simulink model "tank_thermal_sensor_comparison"  (R2025b)
settings: Solver=ode45  StartTime=0.0  StopTime=3600  RelTol=1e-3
libraries: slpidlib x1
settings Model: Creator=maild  LastModifiedBy=maild

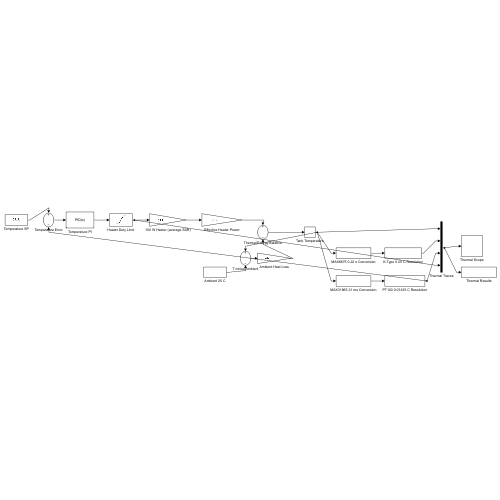
[thumbnail: Simulink's stored preview of the top-level diagram]
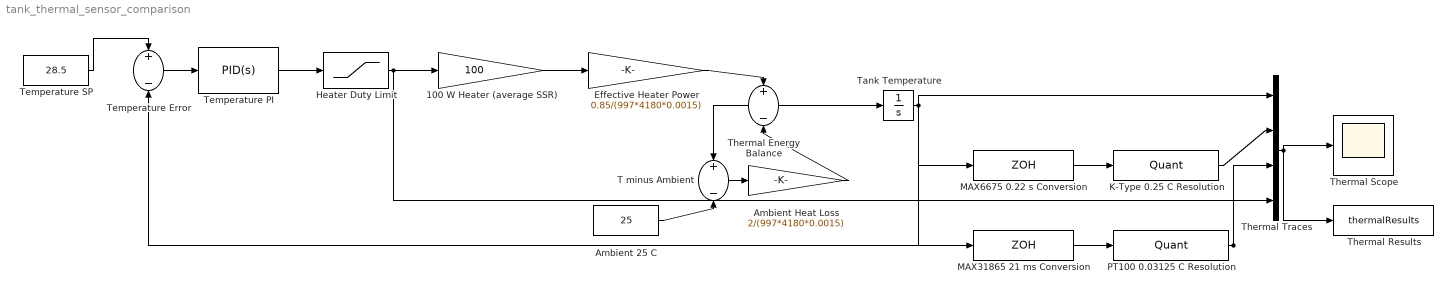
== system tank_thermal_sensor_comparison ==
  100 W Heater (average SSR) : Gain  Gain=100
  Ambient 25 C : Constant  Value=25
  Ambient Heat Loss : Gain  Gain=2/(997*4180*0.0015)
  Effective Heater Power : Gain  Gain=0.85/(997*4180*0.0015)
  Heater Duty Limit : Saturate  UpperLimit=0.10  LowerLimit=0
  K-Type 0.25 C Resolution : Quantizer  QuantizationInterval=0.25
  MAX31865 21 ms Conversion : ZeroOrderHold  SampleTime=0.021
  MAX6675 0.22 s Conversion : ZeroOrderHold  SampleTime=0.22
  PT100 0.03125 C Resolution : Quantizer  QuantizationInterval=0.03125
  T minus Ambient : Sum  Inputs=+-
  Tank Temperature : Integrator  InitialCondition=25
  Temperature Error : Sum  Inputs=+-
  Temperature PI : slpidlib/PID Controller  Controller=PID  Form=Parallel  TimeDomain=Continuous-time  UseExternalTs=off  SampleTime=-1  IntegratorMethod=Forward Euler  FilterMethod=Forward Euler  ControllerParametersSource=internal  P=0.04  I=0.0008  UseKiTs=off  D=0  UseExternalDerivativeSource=off  N=100  UseFilter=on  TunerSelectOption=Transfer Function Based (PID Tuner App)  InitialConditionSource=internal  InitialConditionForIntegrator=0  InitialConditionForFilter=0  DifferentiatorICPrevScaledInput=0  ExternalReset=none  TrackingMode=off  Kt=1  LimitOutput=off  SatLimitsSource=internal  UpperSaturationLimit=inf  LowerSaturationLimit=-inf  LinearizeAsGain=on  AntiWindupMode=none  Kb=1  LimitIntegrator=off  UpperIntegratorSaturationLimit=inf  LowerIntegratorSaturationLimit=-inf  POutMin=[]  POutMax=[]  IOutMin=[]  IOutMax=[]  DOutMin=[]  DOutMax=[]  NOutMin=[]  NOutMax=[]  SumOutMin=[]  SumOutMax=[]  SaturationOutMin=[]  SaturationOutMax=[]  PParamMin=[]  PParamMax=[]  IParamMin=[]  IParamMax=[]  DParamMin=[]  DParamMax=[]  NParamMin=[]  NParamMax=[]  KbParamMin=[]  KbParamMax=[]  KtParamMin=[]  KtParamMax=[]  KbOutMin=[]  KbOutMax=[]  KtOutMin=[]  KtOutMax=[]  IntegratorOutMin=[]  IntegratorOutMax=[]  FilterOutMin=[]  FilterOutMax=[]  SumI1OutMin=[]  SumI1OutMax=[]  SumI2OutMin=[]  SumI2OutMax=[]  SumI3OutMin=[]  SumI3OutMax=[]  SumI4OutMin=[]  SumI4OutMax=[]  SumDOutMin=[]  SumDOutMax=[]  DifferentiatorOutMin=[]  DifferentiatorOutMax=[]  FilterDiffOutCoefMin=[]  FilterDiffOutCoefMax=[]  ReciprocalOutMin=[]  ReciprocalOutMax=[]  SumDenOutMin=[]  SumDenOutMax=[]  SumNumOutMin=[]  SumNumOutMax=[]  DivideOutMin=[]  DivideOutMax=[]  UdiffTsProdOutMin=[]  UdiffTsProdOutMax=[]  NTsProdOutMin=[]  NTsProdOutMax=[]  UintegralTsProdOutMin=[]  UintegralTsProdOutMax=[]  UngainTsProdOutMin=[]  UngainTsProdOutMax=[]  ClampingZeroOutDataTypeStr=Inherit: Inherit via back propagation  ClampingZeroOutMin=[]  ClampingZeroOutMax=[]  FilterDenConstantOutDataTypeStr=Inherit: Inherit via back propagation  FilterDenConstantOutMin=[]  FilterDenConstantOutMax=[]  PCopyOutDataTypeStr=Inherit: Inherit via back propagation  PCopyOutMin=[]  PCopyOutMax=[]  NCopyOutDataTypeStr=Inherit: Inherit via back propagation  NCopyOutMin=[]  NCopyOutMax=[]  IntegratorContinuousStateAttributes=''  IntegratorStateMustResolveToSignalObject=off  IntegratorRTWStateStorageClass=Auto  FilterContinuousStateAttributes=''  FilterStateMustResolveToSignalObject=off  FilterRTWStateStorageClass=Auto  ParallelPVariant=InternalParameters  IdealPVariant=Disabled  IVariant=InternalParameters  DVariant=InternalParameters  IntegratorVariant=Continuous  SatVariant=Disabled  AWVariant=Passthrough  PCopyVariant=Disabled  TRVariant=Disabled  FdbkBlocksVariant=Forward  IdealPFdbkVariant=Disabled  SatFdbkVariant=Disabled  DerivativeFilterVariant=ContFilter  NVariant=InternalParameters  NCopyVariant=Disabled  FilterICVariant=InternalICsFilter  IntegratorICVariant=InternalICs  ExternalResetVariant=Disabled  TRSumVariant=Passthrough  SumFdbkVariant=Disabled  SumVariant=Sum_PID  TsampFilterVariant=InternalTs  TsampNgainVariant=Passthrough  TsampIntegralVariant=Disabled_SignalSpec  ExternalSaturationOutDataTypeStr=Inherit: Same as second input  DerivativeSourceVariant=ErrorSignal  PreIntVariant=InternalPreInt
  Temperature SP : Constant  Value=28.5
  Thermal Energy Balance : Sum  Inputs=+-
  Thermal Results : ToWorkspace  VariableName=thermalResults  SaveFormat=Structure With Time  SampleTime=-1
  Thermal Scope : Scope
  Thermal Traces : Mux
  wires:
  Temperature SP/1 -> Temperature Error/1
  Temperature Error/1 -> Temperature PI/1
  Temperature PI/1 -> Heater Duty Limit/1
  Heater Duty Limit/1 -> 100 W Heater (average SSR)/1, Thermal Traces/4
  100 W Heater (average SSR)/1 -> Effective Heater Power/1
  Effective Heater Power/1 -> Thermal Energy Balance/1
  Tank Temperature/1 -> T minus Ambient/1, MAX6675 0.22 s Conversion/1, MAX31865 21 ms Conversion/1, Thermal Traces/1
  Ambient 25 C/1 -> T minus Ambient/2
  T minus Ambient/1 -> Ambient Heat Loss/1
  Ambient Heat Loss/1 -> Thermal Energy Balance/2
  Thermal Energy Balance/1 -> Tank Temperature/1
  MAX6675 0.22 s Conversion/1 -> K-Type 0.25 C Resolution/1
  MAX31865 21 ms Conversion/1 -> PT100 0.03125 C Resolution/1
  PT100 0.03125 C Resolution/1 -> Temperature Error/2, Thermal Traces/3
  K-Type 0.25 C Resolution/1 -> Thermal Traces/2
  Thermal Traces/1 -> Thermal Scope/1, Thermal Results/1
